simulink model "motor_dynamic_next_fuzzy_pid"  (R2021a)
settings: Solver=VariableStepAuto  StartTime=0.0  StopTime=10  RelTol=1e-3
libraries: fuzblock x2, robotmobilelib x1, simulink x1
settings Model: Creator=THANH DAT  LastModifiedBy=THANH DAT

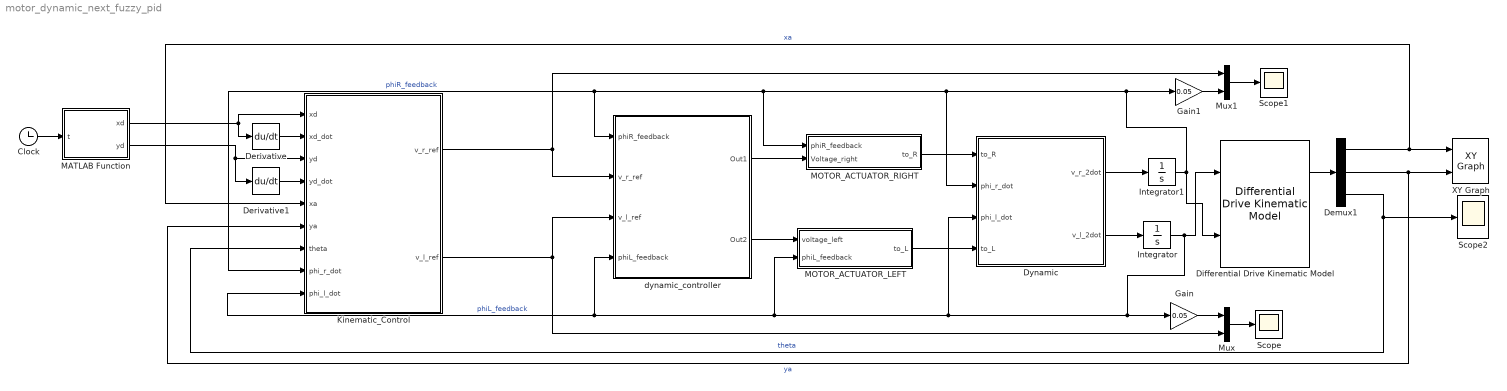
== system motor_dynamic_next_fuzzy_pid ==
  Clock : Clock
  Demux1 : Demux  Outputs=3
  Derivative : Derivative
  Derivative1 : Derivative
  Differential Drive Kinematic Model : robotmobilelib/Differential Drive Kinematic Model  VehicleInputs=Wheel Speeds  WheelRadius=0.05  WheelSpeedRange=[-inf inf]  TrackWidth=0.2  InitialState=[0; 0; 0]  SimulateUsing=Interpreted execution
      settings: SourceProductBaseCode=RO
  Dynamic : Subsystem
  Gain : Gain  Gain=0.05
  Gain1 : Gain  Gain=0.05
  Integrator : Integrator
  Integrator1 : Integrator
  Kinematic_Control : MATLAB Function  TreatAsAtomicUnit=on
  MATLAB Function : MATLAB Function  TreatAsAtomicUnit=on
  MOTOR_ACTUATOR_LEFT : Subsystem
  MOTOR_ACTUATOR_RIGHT : Subsystem
  Mux : Mux  Inputs=2
  Mux1 : Mux  Inputs=2
  Scope : Scope
  Scope1 : Scope
  Scope2 : Scope
  XY Graph : simulink/Sinks/XY Graph  xmin=-10  xmax=10  ymin=-10  ymax=10  st=0.1
  dynamic_controller : Subsystem
  wires:
  Integrator1/1 -> Differential Drive Kinematic Model/2, Dynamic/2(phi_r_dot), Kinematic_Control/8(phi_r_dot), dynamic_controller/1(phiR_feedback), MOTOR_ACTUATOR_RIGHT/1(phiR_feedback), Gain1/1  "phiR_feedback"
  Integrator/1 -> Differential Drive Kinematic Model/1, Gain/1, Dynamic/3(phi_l_dot), Kinematic_Control/9(phi_l_dot), dynamic_controller/4(phiL_feedback), MOTOR_ACTUATOR_LEFT/2(phiL_feedback)  "phiL_feedback"
  Kinematic_Control/1(v_r_ref) -> dynamic_controller/2(v_r_ref), Mux1/1
  Kinematic_Control/2(v_l_ref) -> dynamic_controller/3(v_l_ref), Mux/2
  Mux1/1 -> Scope1/1
  Mux/1 -> Scope/1
  Gain1/1 -> Mux1/2
  Gain/1 -> Mux/1
  dynamic_controller/1(Out1) -> MOTOR_ACTUATOR_RIGHT/2(Voltage_right)
  dynamic_controller/2(Out2) -> MOTOR_ACTUATOR_LEFT/1(voltage_left)
  MOTOR_ACTUATOR_RIGHT/1(to_R) -> Dynamic/1(to_R)
  MOTOR_ACTUATOR_LEFT/1(to_L) -> Dynamic/4(to_L)
  Differential Drive Kinematic Model/1 -> Demux1/1
  Demux1/1 -> Kinematic_Control/5(xa), XY Graph/1  "xa"
  Demux1/2 -> Kinematic_Control/6(ya), XY Graph/2  "ya"
  Demux1/3 -> Scope2/1, Kinematic_Control/7(theta)  "theta"
  Dynamic/1(v_r_2dot) -> Integrator1/1
  Dynamic/2(v_l_2dot) -> Integrator/1
  MATLAB Function/1(xd) -> Kinematic_Control/1(xd), Derivative/1
  MATLAB Function/2(yd) -> Kinematic_Control/3(yd), Derivative1/1
  Derivative/1 -> Kinematic_Control/2(xd_dot)
  Derivative1/1 -> Kinematic_Control/4(yd_dot)
  Clock/1 -> MATLAB Function/1(t)

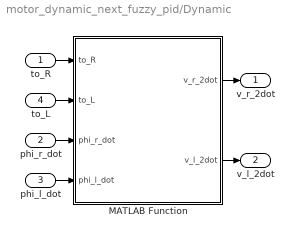
== system motor_dynamic_next_fuzzy_pid/Dynamic ==
  to_R : Inport
  phi_r_dot : Inport  Port=2
  phi_l_dot : Inport  Port=3
  to_L : Inport  Port=4
  MATLAB Function : MATLAB Function  TreatAsAtomicUnit=on
  v_r_2dot : Outport
  v_l_2dot : Outport  Port=2
  wires:
  phi_l_dot/1 -> MATLAB Function/4(phi_l_dot)
  to_L/1 -> MATLAB Function/2(to_L)
  phi_r_dot/1 -> MATLAB Function/3(phi_r_dot)
  MATLAB Function/2(v_l_2dot) -> v_l_2dot/1
  MATLAB Function/1(v_r_2dot) -> v_r_2dot/1
  to_R/1 -> MATLAB Function/1(to_R)

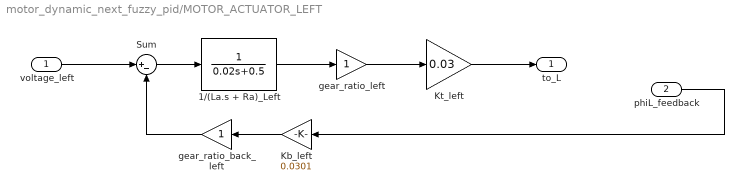
== system motor_dynamic_next_fuzzy_pid/MOTOR_ACTUATOR_LEFT ==
  voltage_left : Inport
  phiL_feedback : Inport  Port=2
  1/(La.s + Ra)_Left : TransferFcn  Denominator=[0.02 0.5]
  Kb_left : Gain  Gain=0.0301
  Kt_left : Gain  Gain=0.03
  Sum : Sum  Inputs=|+-
  gear_ratio_back_left : Gain
  gear_ratio_left : Gain
  to_L : Outport
  wires:
  gear_ratio_left/1 -> Kt_left/1
  1/(La.s + Ra)_Left/1 -> gear_ratio_left/1
  Sum/1 -> 1/(La.s + Ra)_Left/1
  Kt_left/1 -> to_L/1
  Kb_left/1 -> gear_ratio_back_left/1
  phiL_feedback/1 -> Kb_left/1
  voltage_left/1 -> Sum/1
  gear_ratio_back_left/1 -> Sum/2

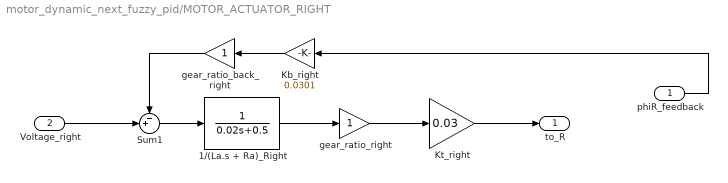
== system motor_dynamic_next_fuzzy_pid/MOTOR_ACTUATOR_RIGHT ==
  phiR_feedback : Inport
  Voltage_right : Inport  Port=2
  1/(La.s + Ra)_Right : TransferFcn  Denominator=[0.02 0.5]
  Kb_right : Gain  Gain=0.0301
  Kt_right : Gain  Gain=0.03
  Sum1 : Sum  Inputs=-+|
  gear_ratio_back_right : Gain
  gear_ratio_right : Gain
  to_R : Outport
  wires:
  Kt_right/1 -> to_R/1
  1/(La.s + Ra)_Right/1 -> gear_ratio_right/1
  gear_ratio_right/1 -> Kt_right/1
  phiR_feedback/1 -> Kb_right/1
  Kb_right/1 -> gear_ratio_back_right/1
  Sum1/1 -> 1/(La.s + Ra)_Right/1
  gear_ratio_back_right/1 -> Sum1/1
  Voltage_right/1 -> Sum1/2

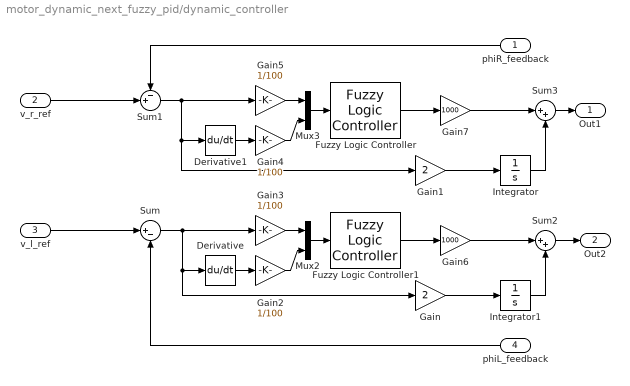
== system motor_dynamic_next_fuzzy_pid/dynamic_controller ==
  phiR_feedback : Inport
  v_r_ref : Inport  Port=2
  v_l_ref : Inport  Port=3
  phiL_feedback : Inport  Port=4
  Derivative : Derivative
  Derivative1 : Derivative
  Fuzzy Logic Controller : fuzblock/Fuzzy Logic  Controller  FIS='fuzzy_logic_op.fis'  OutputSampleNumber=101  DataType=double  FuzzifiedInputs=off  RuleFiringStrengths=off  RuleOutputs=off  AggregatedOutputs=off  SimulateUsing=Interpreted execution  OutOfRangeInputValueMessage=warning  NoRuleFiredMessage=warning  EmptyOutputFuzzySetMessage=warning
  Fuzzy Logic Controller1 : fuzblock/Fuzzy Logic  Controller  FIS='fuzzy_logic_op.fis'  OutputSampleNumber=101  DataType=double  FuzzifiedInputs=off  RuleFiringStrengths=off  RuleOutputs=off  AggregatedOutputs=off  SimulateUsing=Interpreted execution  OutOfRangeInputValueMessage=warning  NoRuleFiredMessage=warning  EmptyOutputFuzzySetMessage=warning
  Gain : Gain  Gain=2
  Gain1 : Gain  Gain=2
  Gain{2..5} (4 alike) : Gain  Gain=1/100
  Gain6 : Gain  Gain=1000
  Gain7 : Gain  Gain=1000
  Integrator : Integrator
  Integrator1 : Integrator
  Mux2 : Mux  Inputs=2
  Mux3 : Mux  Inputs=2
  Sum : Sum  Inputs=|+-
  Sum1 : Sum  Inputs=-+|
  Sum2 : Sum  Inputs=|++
  Sum3 : Sum  Inputs=|++
  Out1 : Outport
  Out2 : Outport  Port=2
  wires:
  Gain4/1 -> Mux3/2
  Mux3/1 -> Fuzzy Logic Controller/1
  phiR_feedback/1 -> Sum1/1
  Gain3/1 -> Mux2/1
  Gain5/1 -> Mux3/1
  Gain2/1 -> Mux2/2
  Sum1/1 -> Gain5/1, Gain1/1, Derivative1/1
  Fuzzy Logic Controller1/1 -> Gain6/1
  Derivative/1 -> Gain2/1
  Mux2/1 -> Fuzzy Logic Controller1/1
  Fuzzy Logic Controller/1 -> Gain7/1
  Derivative1/1 -> Gain4/1
  Sum/1 -> Gain3/1, Gain/1, Derivative/1
  phiL_feedback/1 -> Sum/2
  Gain/1 -> Integrator1/1
  Gain1/1 -> Integrator/1
  Sum3/1 -> Out1/1
  Gain7/1 -> Sum3/1
  Integrator/1 -> Sum3/2
  Sum2/1 -> Out2/1
  Gain6/1 -> Sum2/1
  Integrator1/1 -> Sum2/2
  v_r_ref/1 -> Sum1/2
  v_l_ref/1 -> Sum/1

== matlab function motor_dynamic_next_fuzzy_pid/Kinematic_Control ==
  data: xd input; v_r_ref output; xd_dot input; yd input; yd_dot input; xa input; ya input; theta input; phi_r_dot input; phi_l_dot input; v_l_ref output
function [v_r_ref,v_l_ref] = fcn(xd,xd_dot,yd,yd_dot,xa,ya,theta,phi_r_dot,phi_l_dot)
r = 0.15;
b = 0.3;
a = 0.2;
mG = 10; 
mW = 2; 
IG = 4; 
ID = 0.05; 
IW = 0.1;
C_2 = 2;
error_x = xd-xa;
error_y = yd-ya;

v = [phi_r_dot;
     phi_l_dot;];
 
D_dot_matrix = [xd_dot;yd_dot];

T_matrix = [cos(theta), sin(theta);
     -sin(theta), cos(theta);];
ep = T_matrix*[error_x;
        error_y;];
ep1 = ep(1,1);
ep2 = ep(2,1);

h_matrix = [(ep2/b -1)*(r/2), -(ep2/b + 1)*(r/2);
            -(ep1*r)/(2*b), (ep1*r)/(2*b)       ;];
        

v1 = -inv(h_matrix)*T_matrix*D_dot_matrix;
v2 = -inv(h_matrix)*C_2*ep; 

v_ref = v1+v2; 

v_r_ref = v_ref(1,1);
v_l_ref = v_ref(2,1);

== matlab function motor_dynamic_next_fuzzy_pid/Dynamic/MATLAB Function ==
  data: to_R input; v_r_2dot output; to_L input; phi_r_dot input; phi_l_dot input; v_l_2dot output
function [v_r_2dot, v_l_2dot]   = dynamic(to_R,to_L, phi_r_dot, phi_l_dot)
%Declaration
r = 0.15;
b = 0.3;
a = 0.2;
mG = 10; 
mW = 2; 
IG = 4; 
ID = 0.05; 
IW = 0.1;
I_matrix = [0, 1;
          -1, 0;];

m11 = mG*((r^2)/4 + (a*r^2)/(4*b^2)) + (r^2/(4*b^2))*(IG + 2*ID) + 2*mW*r^2 + IW;
m12 = mG*((r^2)/4 - ((a^2)*(r^2))/(4*b^2)) - (r^2/(4*b^2))*(IG + 2*ID);
m22 = m11;
m21 = m12; 

omega = r*(phi_r_dot - phi_l_dot)/(2*b);

v = [phi_r_dot;
     phi_l_dot;];

M = [m11, m12;
     m21, m22;];

B = mG*(r^2/(2*b))*omega*I_matrix ;

to = [to_R;
      to_L;]; 

v_dot = -(inv(M))*B*v + (inv(M))*to; 

v_r_2dot = v_dot(1,1);
v_l_2dot = v_dot(2,1);

== matlab function motor_dynamic_next_fuzzy_pid/MATLAB Function ==
  data: t input; xd output; yd output
function [xd,yd] = fcn(t)
xd = 3;
yd = 3;
